simulink model "cic"  (R2014a)
settings: Solver=VariableStepDiscrete  StartTime=0.0  StopTime=0.1  RelTol=1e-3
libraries: dspsigops x1
settings Model: Creator=Yin  LastModifiedBy=Yin

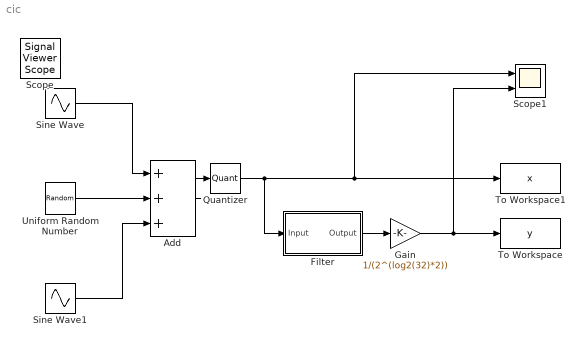
== system cic ==
  Add : Sum  Inputs=+++
  Filter : Subsystem  Tag=FilterWizardSubSystem
      settings: ErrorFcn=dspFilterRealizedInBasicElemsAlgLoopErrFcnCallback
  Gain : Gain  Gain=1/(2^(log2(32)*2))
  Quantizer : Quantizer  QuantizationInterval=1
  Scope1 : Scope  NumInputPorts=2
      settings: TimeRange=0.1  YMin=-2250~-2e+06  YMax=2250~2e+06
  Sine Wave : Sin  Amplitude=2^10  Frequency=2*pi*0.1e3  SampleTime=1/200e3
  Sine Wave1 : Sin  Amplitude=2^6  Frequency=2*pi*1e3  SampleTime=1/200e3
  To Workspace : ToWorkspace  VariableName=y  SampleTime=-1
  To Workspace1 : ToWorkspace  VariableName=x  SampleTime=-1
  Uniform Random Number : UniformRandomNumber  Minimum=-2^7  Maximum=+2^7  SampleTime=1/50e3
  Scope : SignalViewerScope  IOType=viewer  RefreshTime=0.035000
  wires:
  Quantizer/1 -> Scope1/1, To Workspace1/1, Filter/1(Input)
  Sine Wave/1 -> Add/1
  Uniform Random Number/1 -> Add/2
  Add/1 -> Quantizer/1
  Sine Wave1/1 -> Add/3
  Filter/1(Output) -> Gain/1
  Gain/1 -> Scope1/2, To Workspace/1

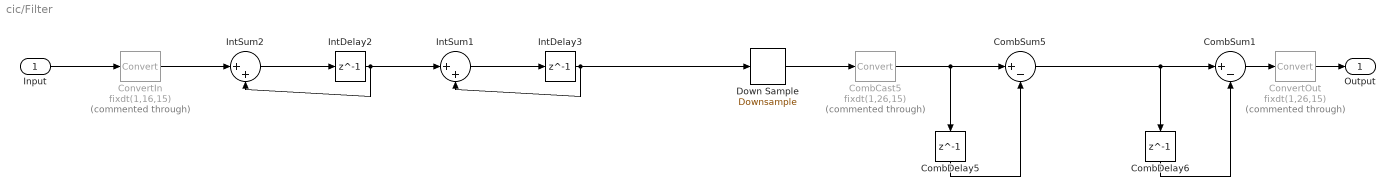
== system cic/Filter ==
  Input : Inport
  CombCast5 : DataTypeConversion  Commented=through  OutDataTypeStr=fixdt(1,26,15)
  CombDelay5 : Delay  DelayLength=1  InitialCondition=0
  CombDelay6 : Delay  DelayLength=1  InitialCondition=0
  CombSum1 : Sum  Inputs=|+-
  CombSum5 : Sum  Inputs=|+-
  ConvertIn : DataTypeConversion  Commented=through  OutDataTypeStr=fixdt(1,16,15)  RndMeth=Nearest  SaturateOnIntegerOverflow=on
  ConvertOut : DataTypeConversion  Commented=through  OutDataTypeStr=fixdt(1,26,15)
  Down Sample : dspsigops/Downsample  N=32  phase=0  RateOptions=Allow multirate processing  smode=Allow multirate  fmode=Maintain input frame size  ic=0
  IntDelay2 : Delay  DelayLength=1  InitialCondition=0
  IntDelay3 : Delay  DelayLength=1  InitialCondition=0
  IntSum1 : Sum  Inputs=|++
  IntSum2 : Sum  Inputs=|++
  Output : Outport
  wires:
  Input/1 -> ConvertIn/1
  ConvertIn/1 -> IntSum2/1
  IntSum2/1 -> IntDelay2/1
  IntDelay2/1 -> IntSum1/1, IntSum2/2
  IntSum1/1 -> IntDelay3/1
  IntDelay3/1 -> IntSum1/2, Down Sample/1
  Down Sample/1 -> CombCast5/1
  CombSum5/1 -> CombSum1/1, CombDelay6/1
  CombDelay5/1 -> CombSum5/2
  CombCast5/1 -> CombSum5/1, CombDelay5/1
  CombSum1/1 -> ConvertOut/1
  CombDelay6/1 -> CombSum1/2
  ConvertOut/1 -> Output/1
